simulink model "sedemo_rtos_dependent_tasks"  (Simulink 7.5)
settings: Solver=VariableStepDiscrete  StartTime=0.0  StopTime=15  MaxStep=inf  RelTol=1e-3
undefined symbols (not defined in the file or in its folder): des_figposition
libraries: simeventssink1 x8, simeventsgenerators1 x6, simeventsrouting1 x3, simeventsattributes2 x3, simeventsserver1 x1, simeventsinfo x1, simeventstranslate1 x1, simeventsqueue1 x1
settings Model: Creator=The MathWorks Inc.  ExtModeAutoUpdateStatusClock=off
settings DataIOCC: SaveOutput=off  SaveTime=off
settings OptimizationCC: InitFltsAndDblsToZero=on
settings DebuggingCC: AlgebraicLoopMsg=error  SignalResolutionControl=TryResolveAllWithWarning  SolverPrmCheckMsg=none  MultiTaskDSMMsg=warning  MultiTaskCondExecSysMsg=none  StrictBusMsg=Warning
settings RTWCC: IncludeERTFirstTime=on
settings GRTTargetCC: TargetFcnLib=ansi_tfl_tmw_new.mat
settings SimEventsCC: propDiagAttribOutput=1  propDiagFcnCallOutput=1  propDiagStatOutput=0

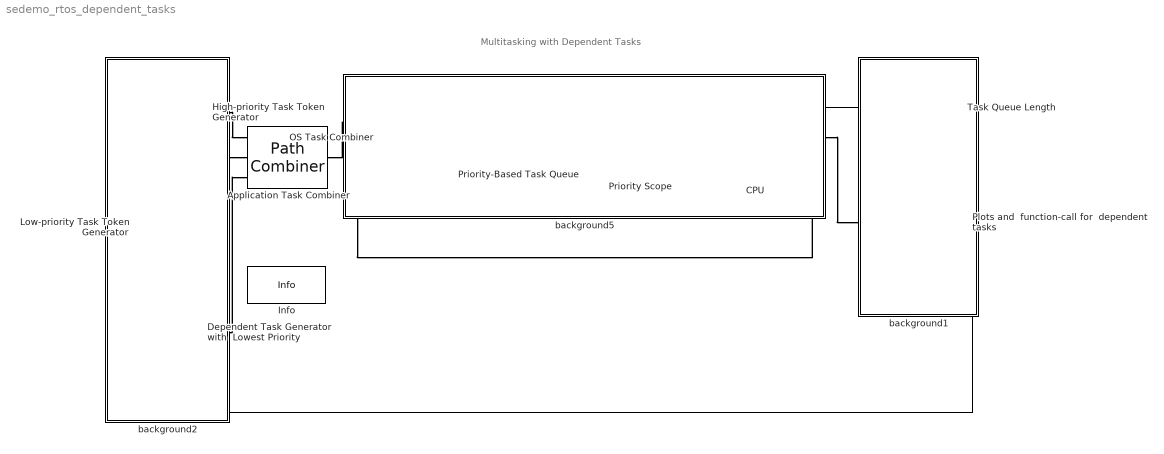
== system sedemo_rtos_dependent_tasks ==
  note: Multitasking with Dependent Tasks
  Application Task Combiner : simeventsrouting1/Path Combiner  Priority=1  SystemSampleTime=-1  NumberInputPorts=3  InputPortPrecedence=IN1 port  InitialSeed=45675  SpecifyEventPriority=off  PriorityPathCombinerPortPrecedenceSelection=4100  StatNumberDeparted=Off  StatLastArrivalPort=Off  EvaluatedNumPorts=3
  CPU : simeventsserver1/Single Server  Priority=1  SystemSampleTime=-1  ServiceTimeFrom=Attribute  ServiceTime=0.5  AttributeName=TaskExecTime  PriorityServiceCompletion=500  PermitPreemption=on  SortingAttributeName=PriorityAttributeName  SortingDirection=Ascending  WriteToAttribute=on  ResidualAttributeName=TaskExecTime  CreateAttribute=off  EnableTOPort=off  StatNumberDeparted=Off  StatNumberInBlock=Off  StatNumberPreempted=Off  StatPendingEntity=Off  StatAverageWait=Off  StatUtilization=Off  StatNumberTimedout=Off
  Dependent Task Generator with  Lowest Priority : Subsystem
  High-priority Task Token Generator : Subsystem
  Info : simeventsinfo/Info  SystemSampleTime=-1
  Low-priority Task Token Generator : Subsystem
  OS Task Combiner : simeventsrouting1/Path Combiner  Priority=1  SystemSampleTime=-1  NumberInputPorts=2  InputPortPrecedence=IN1 port  InitialSeed=45675  SpecifyEventPriority=off  PriorityPathCombinerPortPrecedenceSelection=4100  StatNumberDeparted=Off  StatLastArrivalPort=Off  EvaluatedNumPorts=2
  Plots and  function-call for  dependent tasks : Subsystem
  Priority Scope : simeventssink1/Attribute Scope  Priority=1  SystemSampleTime=-1  PlotType=Stair  InputType=Attribute  NumInputs=1  AttributeNameY=PriorityAttributeName  XInputOptionSignal=Event time  XInputOptionEntity=Event time  AttributeNameX=Count  EnableEntityOutport=on  XMin=0  XMax=15.5  XLimitExceededOption=Stretch axis limits  YLimitExceededOption=Stretch axis limits  AxisGrid=on  AxisLegend=off  LineDisables=""  LineColors=b  LineStyles=-  LineMarkers=.  OpenScopeAtSimStart=on  Title=Priority Value for Tasks  YLabel=Priority  XLabel=Time  FigurePosition=des_figposition([2 15 24 20])  AxisZoom=off  DataStoreOption=Limited  DataPointsLimit=10000  StatNumberArrived=Off  ShowCountPlotted=off  ShowToolbar=off
      settings: YMin=0  YMax=3
  Priority-Based Task Queue : simeventsqueue1/Priority Queue  Priority=1  SystemSampleTime=-1  Capacity=inf  SortingAttributeName=PriorityAttributeName  SortingDirection=Ascending  EnableTOPort=off  StatNumberDeparted=Off  StatNumberInBlock=On  StatPendingEntity=Off  StatAverageWait=Off  StatAverageQueueLength=Off  StatNumberTimedout=Off
  Task Queue Length : simeventssink1/Signal Scope  Priority=1  SystemSampleTime=-1  PlotType=Stair  InputType=Signal  NumInputs=1  AttributeNameY=Count  XInputOptionSignal=Event time  XInputOptionEntity=Event time  AttributeNameX=Count  EnableEntityOutport=on  XMin=0  XMax=15  XLimitExceededOption=Stretch axis limits  YLimitExceededOption=Stretch axis limits  AxisGrid=on  AxisLegend=off  LineDisables=""  LineColors=b  LineStyles=-  LineMarkers=.  OpenScopeAtSimStart=on  Title=Queue Length  YLabel=Number of Tasks  XLabel=Time  FigurePosition=des_figposition([26 15 24 20])  AxisZoom=off  DataStoreOption=Limited  DataPointsLimit=10000  StatNumberArrived=Off  ShowCountPlotted=off  ShowToolbar=off
      settings: YMin=0  YMax=4
  background1 : Subsystem
      mask Display: disp('')
  background2 : Subsystem
      mask Display: disp('')
  background5 : Subsystem
      mask Display: disp('')
  wires:
  Priority-Based Task Queue/1 -> Task Queue Length/1
  Plots and  function-call for  dependent tasks/1(Out1) -> Dependent Task Generator with  Lowest Priority/1(In1)
  connections:
  CPU/RConn1 -- Plots and  function-call for  dependent tasks/LConn1
  OS Task Combiner/RConn1 -- Priority-Based Task Queue/LConn1
  OS Task Combiner/LConn2 -- CPU/RConn2
  High-priority Task Token Generator/RConn1 -- Application Task Combiner/LConn1
  Low-priority Task Token Generator/RConn1 -- Application Task Combiner/LConn2
  Priority Scope/LConn1 -- Priority-Based Task Queue/RConn1
  CPU/LConn1 -- Priority Scope/RConn1
  Application Task Combiner/RConn1 -- OS Task Combiner/LConn1
  Dependent Task Generator with  Lowest Priority/RConn1 -- Application Task Combiner/LConn3

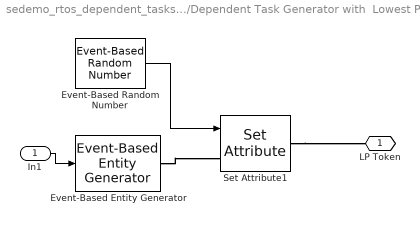
== system sedemo_rtos_dependent_tasks/Dependent Task Generator with  Lowest Priority ==
  In1 : Inport  OutDataType=sfix(16)  OutScaling=2^0
  Event-Based Entity Generator : simeventsgenerators1/Entity Generators/Event-Based Entity Generator  Priority=1  DialogController=des_ddg_create  DialogControllerArgs=DataTag3  SystemSampleTime=-1  GenerateEntitiesUpon=Function call from port fcn  SignalEdgeType=Rising  SpecifyEventPriority=off  PriorityEntityGeneration=300  GenerateEntityAtSimulationStart=on  AllowBlocking=on  ResponseDuringBlockage=Discard generated entities  EntityType=Standard  StatNumberDeparted=Off  StatPendingEntity=Off  StatAverageIntergenerationTime=Off
  Event-Based Random Number : simeventsgenerators1/Signal Generators/Event-Based Random Number  SystemSampleTime=-1  distribution=Uniform  meanExp=2  minUnif=0.05  maxUnif=0.05  pOneBern=0.25  pSuccessBino=0.5  numTrialBino=1  meanNorm=0  stdNorm=1  minTri=1  maxTri=3  modeTri=2  thresholdLogn=0  scaleLogn=1  shapeLogn=1  pSuccessGeo=0.5  meanPoiss=1  thresholdLogl=0  scaleLogl=1  thresholdGam=0  scaleGam=1  shapeGam=1  minBeta=0  maxBeta=1  shape1Beta=1  shape2Beta=1  minUnid=0  maxUnid=1  numValueUnid=2  thresholdWbl=0  scaleWbl=1  shapeWbl=1  valueVecCont=[0 1]  cdfVecCont=[0 1]  valueVecDisc=[0 1]  probVecDisc=[0.5 0.5]  seed=7507  IsProcessed=on  isConnected=1
  Set Attribute1 : simeventsattributes2/Set Attribute  Priority=1  DialogController=des_ddg_create  DialogControllerArgs=DataTag5  SystemSampleTime=-1  AttributeFrom=Dialog|Signal port  AttributeName=PriorityAttributeName|TaskExecTime  AttributeTreatAsVector=1|1  AttributeValue=3|1  AttributeCreate=on  StatNumberDeparted=Off  EvaluatedAttributeValue={3;[]}
  LP Token : PMIOPort  Port=1  Side=Right
  wires:
  Event-Based Random Number/1 -> Set Attribute1/1
  In1/1 -> Event-Based Entity Generator/1
  connections:
  Set Attribute1/RConn1 -- LP Token/RConn1
  Event-Based Entity Generator/RConn1 -- Set Attribute1/LConn1

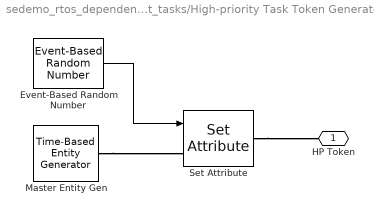
== system sedemo_rtos_dependent_tasks/High-priority Task Token Generator ==
  Event-Based Random Number : simeventsgenerators1/Signal Generators/Event-Based Random Number  SystemSampleTime=-1  distribution=Uniform  meanExp=0.9  minUnif=0.25  maxUnif=0.3  pOneBern=0.25  pSuccessBino=0.5  numTrialBino=1  meanNorm=0  stdNorm=1  minTri=1  maxTri=3  modeTri=2  thresholdLogn=0  scaleLogn=1  shapeLogn=1  pSuccessGeo=0.5  meanPoiss=1  thresholdLogl=0  scaleLogl=1  thresholdGam=0  scaleGam=1  shapeGam=1  minBeta=0  maxBeta=1  shape1Beta=1  shape2Beta=1  minUnid=0  maxUnid=1  numValueUnid=2  thresholdWbl=0  scaleWbl=1  shapeWbl=1  valueVecCont=[0 1]  cdfVecCont=[0 1]  valueVecDisc=[0 1]  probVecDisc=[0.5 0.5]  seed=25899  IsProcessed=on  isConnected=1
  Master Entity Gen : simeventsgenerators1/Entity Generators/Time-Based Entity Generator  Priority=1  DialogController=des_ddg_create  DialogControllerArgs=DataTag7  SystemSampleTime=-1  GenerateEntitiesUpon=Intergeneration time from dialog  Distribution=Constant  Minimum=0.75  Maximum=1  Mean=1  InitialSeed=12345  Period=1  PriorityEntityGeneration=200  GenerateEntityAtSimulationStart=on  ResponseWhenBlocked=Pause generation  ResponseWhenUnblocked=Immediate restart  EntityType=Standard  StatNumberDeparted=Off  StatPendingEntity=Off  StatAverageIntergenerationTime=Off
  Set Attribute : simeventsattributes2/Set Attribute  Priority=1  DialogController=des_ddg_create  DialogControllerArgs=DataTag9  SystemSampleTime=-1  AttributeFrom=Dialog|Signal port  AttributeName=PriorityAttributeName|TaskExecTime  AttributeTreatAsVector=1|1  AttributeValue=1|1  AttributeCreate=on  StatNumberDeparted=Off  EvaluatedAttributeValue={1;[]}
  HP Token : PMIOPort  Port=1  Side=Right
  wires:
  Event-Based Random Number/1 -> Set Attribute/1
  connections:
  Master Entity Gen/RConn1 -- Set Attribute/LConn1
  Set Attribute/RConn1 -- HP Token/RConn1

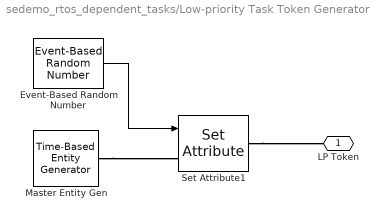
== system sedemo_rtos_dependent_tasks/Low-priority Task Token Generator ==
  Event-Based Random Number : simeventsgenerators1/Signal Generators/Event-Based Random Number  SystemSampleTime=-1  distribution=Uniform  meanExp=2  minUnif=0.3  maxUnif=0.35  pOneBern=0.25  pSuccessBino=0.5  numTrialBino=1  meanNorm=0  stdNorm=1  minTri=1  maxTri=3  modeTri=2  thresholdLogn=0  scaleLogn=1  shapeLogn=1  pSuccessGeo=0.5  meanPoiss=1  thresholdLogl=0  scaleLogl=1  thresholdGam=0  scaleGam=1  shapeGam=1  minBeta=0  maxBeta=1  shape1Beta=1  shape2Beta=1  minUnid=0  maxUnid=1  numValueUnid=2  thresholdWbl=0  scaleWbl=1  shapeWbl=1  valueVecCont=[0 1]  cdfVecCont=[0 1]  valueVecDisc=[0 1]  probVecDisc=[0.5 0.5]  seed=811  IsProcessed=on  isConnected=1
  Master Entity Gen : simeventsgenerators1/Entity Generators/Time-Based Entity Generator  Priority=1  DialogController=des_ddg_create  DialogControllerArgs=DataTag11  SystemSampleTime=-1  GenerateEntitiesUpon=Intergeneration time from dialog  Distribution=Uniform  Minimum=0.5  Maximum=0.7  Mean=1  InitialSeed=12345  Period=3  PriorityEntityGeneration=200  GenerateEntityAtSimulationStart=on  ResponseWhenBlocked=Pause generation  ResponseWhenUnblocked=Immediate restart  EntityType=Standard  StatNumberDeparted=Off  StatPendingEntity=Off  StatAverageIntergenerationTime=Off
  Set Attribute1 : simeventsattributes2/Set Attribute  Priority=1  DialogController=des_ddg_create  DialogControllerArgs=DataTag13  SystemSampleTime=-1  AttributeFrom=Dialog|Signal port  AttributeName=PriorityAttributeName|TaskExecTime  AttributeTreatAsVector=1|1  AttributeValue=2|1  AttributeCreate=on  StatNumberDeparted=Off  EvaluatedAttributeValue={2;[]}
  LP Token : PMIOPort  Port=1  Side=Right
  wires:
  Event-Based Random Number/1 -> Set Attribute1/1
  connections:
  Master Entity Gen/RConn1 -- Set Attribute1/LConn1
  Set Attribute1/RConn1 -- LP Token/RConn1

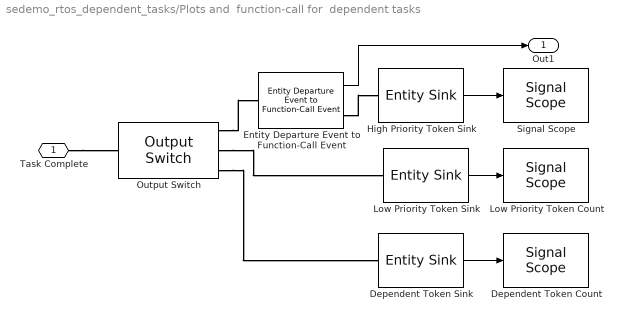
== system sedemo_rtos_dependent_tasks/Plots and  function-call for  dependent tasks ==
  Dependent Token Count : simeventssink1/Signal Scope  Priority=1  SystemSampleTime=-1  PlotType=Stair  InputType=Signal  NumInputs=1  AttributeNameY=Count  XInputOptionSignal=Event time  XInputOptionEntity=Event time  AttributeNameX=Count  EnableEntityOutport=on  XMin=-0.146543987284931  XMax=14.8009427157781  XLimitExceededOption=Stretch axis limits  YLimitExceededOption=Stretch axis limits  AxisGrid=on  AxisLegend=off  LineDisables=""  LineColors=b  LineStyles=-  LineMarkers=.  OpenScopeAtSimStart=on  Title=Dependent Tasks Completed  YLabel=Number of Tasks  XLabel=Time  FigurePosition=des_figposition([74 40 24 20])  AxisZoom=off  DataStoreOption=Limited  DataPointsLimit=10000  StatNumberArrived=Off  ShowCountPlotted=off  ShowToolbar=off
      settings: YMin=-0.15  YMax=15.15
  Dependent Token Sink : simeventssink1/Entity Sink  Priority=1  SystemSampleTime=-1  AvailableForArrivals=on  StatNumberArrived=On
  Entity Departure Event to Function-Call Event : simeventstranslate1/Entity Departure Event to Function-Call Event  Priority=1  SystemSampleTime=-1  TimingFunctionCallF1=After entity departure  EnableE1Port=off  EnableF2Port=off  TimingFunctionCallF2=Before entity departure  EnableE2Port=off  StatNumberDeparted=Off  StatNumberF1Calls=Off  StatNumberF2Calls=Off  IsInsideAFB=off
  "High Priority Token Sink " : simeventssink1/Entity Sink  Priority=1  SystemSampleTime=-1  AvailableForArrivals=on  StatNumberArrived=On
  Low Priority Token Count : simeventssink1/Signal Scope  Priority=1  SystemSampleTime=-1  PlotType=Stair  InputType=Signal  NumInputs=1  AttributeNameY=Count  XInputOptionSignal=Event time  XInputOptionEntity=Event time  AttributeNameX=Count  EnableEntityOutport=on  XMin=0  XMax=15  XLimitExceededOption=Stretch axis limits  YLimitExceededOption=Stretch axis limits  AxisGrid=on  AxisLegend=off  LineDisables=""  LineColors=b  LineStyles=-  LineMarkers=.  OpenScopeAtSimStart=on  Title=Low Priority Tasks Completed  YLabel=Number of Tasks  XLabel=Time  FigurePosition=des_figposition([50 15 24 20])  AxisZoom=off  DataStoreOption=Limited  DataPointsLimit=10000  StatNumberArrived=Off  ShowCountPlotted=off  ShowToolbar=off
      settings: YMin=0  YMax=30
  Low Priority Token Sink : simeventssink1/Entity Sink  Priority=1  SystemSampleTime=-1  AvailableForArrivals=on  StatNumberArrived=On
  Output Switch : simeventsrouting1/Output Switch  Priority=1  SystemSampleTime=-1  NumberOutputPorts=3  SwitchingCriterion=From attribute  InitialSeed=34567  AttributeName=PriorityAttributeName  InitialConditionsOpt=off  InitialConditions=1  EntityBufferOpt=off  SpecifyEventPriority=off  PriorityOutputSwitchSelectPort=4100  TimeoutPortOpt=off  StatNumberDeparted=Off  StatNumberTimedOut=Off  StatPendingEntity=Off  StatLastDeparturePort=Off  EvaluatedNumPorts=3
  Signal Scope : simeventssink1/Signal Scope  Priority=1  SystemSampleTime=-1  PlotType=Stair  InputType=Signal  NumInputs=1  AttributeNameY=Count  XInputOptionSignal=Event time  XInputOptionEntity=Event time  AttributeNameX=Count  EnableEntityOutport=on  XMin=-0.142702821880508  XMax=14.4129850099314  XLimitExceededOption=Stretch axis limits  YLimitExceededOption=Stretch axis limits  AxisGrid=on  AxisLegend=off  LineDisables=""  LineColors=b  LineStyles=-  LineMarkers=.  OpenScopeAtSimStart=on  Title=High Priority Tasks Completed  YLabel=Number of Tasks  XLabel=Time  FigurePosition=des_figposition([74 15 24 20])  AxisZoom=off  DataStoreOption=Limited  DataPointsLimit=10000  StatNumberArrived=Off  ShowCountPlotted=off  ShowToolbar=off
      settings: YMin=-0.15  YMax=15.15
  Task Complete : PMIOPort  Port=1  Side=Left
  Out1 : Outport  OutDataType=sfix(16)  OutScaling=2^0
  wires:
  Low Priority Token Sink/1 -> Low Priority Token Count/1
  "High Priority Token Sink "/1 -> Signal Scope/1
  Entity Departure Event to Function-Call Event/1 -> Out1/1
  Dependent Token Sink/1 -> Dependent Token Count/1
  connections:
  Task Complete/RConn1 -- Output Switch/LConn1
  Output Switch/RConn2 -- Low Priority Token Sink/LConn1
  Output Switch/RConn1 -- Entity Departure Event to Function-Call Event/LConn1
  Entity Departure Event to Function-Call Event/RConn1 -- "High Priority Token Sink "/LConn1
  Output Switch/RConn3 -- Dependent Token Sink/LConn1

== system sedemo_rtos_dependent_tasks/background1 ==

== system sedemo_rtos_dependent_tasks/background2 ==

== system sedemo_rtos_dependent_tasks/background5 ==
